simulink model "vx_vy_fixed_fusion_v2_5c_compile_harness"  (R2024a)
settings: Solver=FixedStepDiscrete  StartTime=0  StopTime=0.1  FixedStep=0.001  RelTol=1e-3
model workspace (MAT data in the model file):
  vy_v17_mode_code = 20
undefined symbols (not defined in the file or in its folder): vy_dynamic_ekf_v1_17
libraries: simulink x3
Description:
  | V2.5-C estimator-only compile harness. No CarSim or plant. Fusion weights [1/3 1/3 1/3] are TEST-ONLY, NOT SELECTED, NOT TUNED, NOT FROZEN. F feedback valid is fixed false and Vy_FW is not fed back.
settings Model: Creator=21180  LastModifiedBy=21180

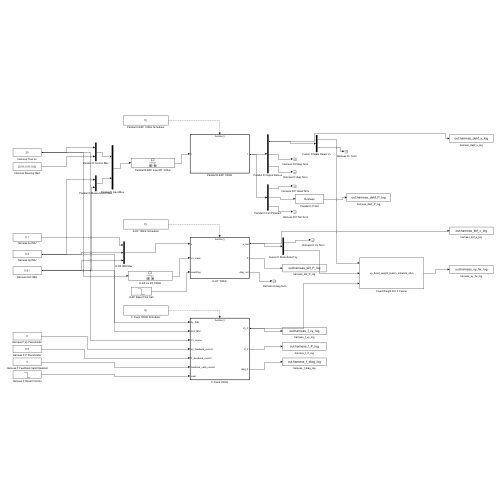
[thumbnail: Simulink's stored preview of the top-level diagram]
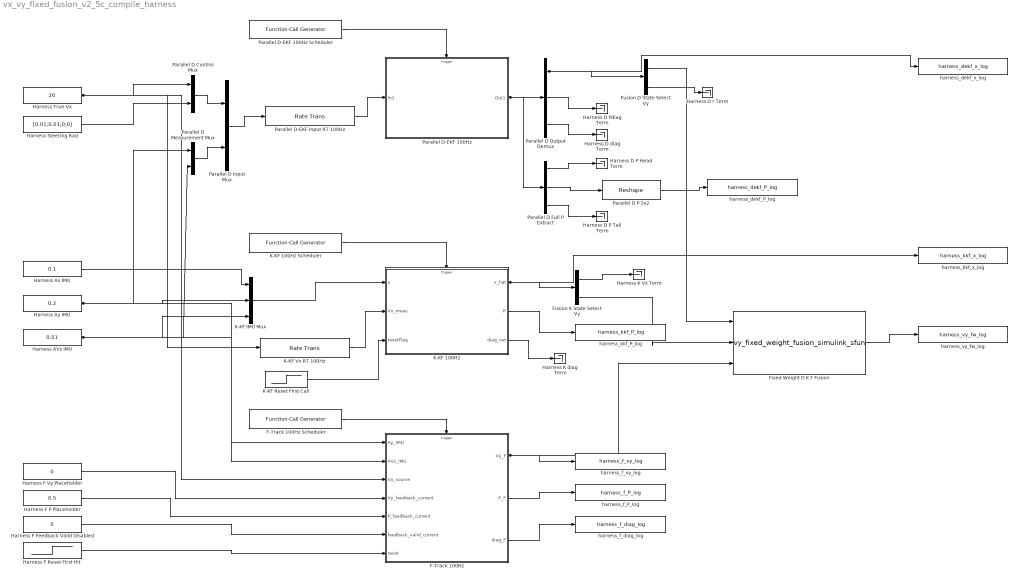
== system vx_vy_fixed_fusion_v2_5c_compile_harness ==
  F-Track 100Hz : Subsystem  TreatAsAtomicUnit=on
  F-Track 100Hz Scheduler : simulink/Ports & Subsystems/Function-Call Generator  sample_time=0.01  numberOfIterations=1  DisallowWideOutput=off
  Fixed Weight D K F Fusion : M-S-Function  FunctionName=vy_fixed_weight_fusion_simulink_sfun  Parameters=1/3,1/3,1/3
  Fusion D State Select Vy : Demux  Outputs=2
  Fusion K State Select Vy : Demux  Outputs=2
  Harness AVz IMU : Constant  Value=0.01  OutDataTypeStr=double  SampleTime=0.01
  Harness Ax IMU : Constant  Value=0.1  OutDataTypeStr=double  SampleTime=0.01
  Harness Ay IMU : Constant  Value=0.2  OutDataTypeStr=double  SampleTime=0.01
  Harness D P Head Term : Terminator
  Harness D P Tail Term : Terminator
  Harness D Pdiag Term : Terminator
  Harness D diag Term : Terminator
  Harness D r Term : Terminator
  Harness F Feedback Valid Disabled : Constant  Value=0  OutDataTypeStr=double  SampleTime=0.01
  Harness F P Placeholder : Constant  Value=0.5  OutDataTypeStr=double  SampleTime=0.01
  Harness F Reset First Hit : Step  Time=0.01  Before=1  After=0  SampleTime=0.01
  Harness F Vy Placeholder : Constant  Value=0  OutDataTypeStr=double  SampleTime=0.01
  Harness K Vx Term : Terminator
  Harness K diag Term : Terminator
  Harness Steering Rad : Constant  Value=[0.01;0.01;0;0]  OutDataTypeStr=double  SampleTime=0.01
  Harness True Vx : Constant  Value=20  OutDataTypeStr=double  SampleTime=0.001
  K-KF 100Hz : Subsystem  TreatAsAtomicUnit=on
  K-KF 100Hz Scheduler : simulink/Ports & Subsystems/Function-Call Generator  sample_time=0.01  numberOfIterations=1  DisallowWideOutput=off
  K-KF IMU Mux : Mux  Inputs=3
  K-KF Reset First Call : Step  Time=0.01  Before=1  After=0  SampleTime=0.01
  K-KF Vx RT 100Hz : RateTransition  OutPortSampleTime=0.01
  Parallel D Control Mux : Mux  Inputs=[1 4]
  Parallel D Full P Extract : Demux  Outputs=[45 4 20]
  Parallel D Input Mux : Mux  Inputs=[5 2]
  Parallel D Measurement Mux : Mux  Inputs=2
  Parallel D Output Demux : Demux  Outputs=[2 2 65]
  Parallel D P 2x2 : Reshape  OutputDimensionality=Customize  OutputDimensions=[2 2]
  Parallel D-EKF 100Hz : Subsystem  TreatAsAtomicUnit=on
  Parallel D-EKF 100Hz Scheduler : simulink/Ports & Subsystems/Function-Call Generator  sample_time=0.01  numberOfIterations=1  DisallowWideOutput=off
  Parallel D-EKF Input RT 100Hz : RateTransition  OutPortSampleTime=0.01
  harness_dekf_P_log : ToWorkspace  VariableName=harness_dekf_P_log  SaveFormat=Timeseries  SampleTime=-1
  harness_dekf_x_log : ToWorkspace  VariableName=harness_dekf_x_log  SaveFormat=Timeseries  SampleTime=-1
  harness_f_P_log : ToWorkspace  VariableName=harness_f_P_log  SaveFormat=Timeseries  SampleTime=-1
  harness_f_diag_log : ToWorkspace  VariableName=harness_f_diag_log  SaveFormat=Timeseries  SampleTime=-1
  harness_f_vy_log : ToWorkspace  VariableName=harness_f_vy_log  SaveFormat=Timeseries  SampleTime=-1
  harness_kkf_P_log : ToWorkspace  VariableName=harness_kkf_P_log  SaveFormat=Timeseries  SampleTime=-1
  harness_kkf_x_log : ToWorkspace  VariableName=harness_kkf_x_log  SaveFormat=Timeseries  SampleTime=-1
  harness_vy_fw_log : ToWorkspace  VariableName=harness_vy_fw_log  SaveFormat=Timeseries  SampleTime=-1
  wires:
  Harness True Vx/1 -> Parallel D Control Mux/1, K-KF Vx RT 100Hz/1, F-Track 100Hz/3(Vx_source)
  Harness Steering Rad/1 -> Parallel D Control Mux/2
  Harness Ay IMU/1 -> Parallel D Measurement Mux/1, K-KF IMU Mux/2, F-Track 100Hz/1(Ay_IMU)
  Harness AVz IMU/1 -> Parallel D Measurement Mux/2, K-KF IMU Mux/3, F-Track 100Hz/2(AVz_IMU)
  Parallel D Control Mux/1 -> Parallel D Input Mux/1
  Parallel D Measurement Mux/1 -> Parallel D Input Mux/2
  Parallel D Input Mux/1 -> Parallel D-EKF Input RT 100Hz/1
  Parallel D-EKF Input RT 100Hz/1 -> Parallel D-EKF 100Hz/1(In1)
  Parallel D-EKF 100Hz Scheduler/1 -> Parallel D-EKF 100Hz/Trigger
  Parallel D-EKF 100Hz/1(Out1) -> Parallel D Output Demux/1, Parallel D Full P Extract/1
  Parallel D Full P Extract/2 -> Parallel D P 2x2/1
  Harness Ax IMU/1 -> K-KF IMU Mux/1
  K-KF IMU Mux/1 -> K-KF 100Hz/1(u)
  K-KF Vx RT 100Hz/1 -> K-KF 100Hz/2(Vx_meas)
  K-KF Reset First Call/1 -> K-KF 100Hz/3(resetFlag)
  K-KF 100Hz Scheduler/1 -> K-KF 100Hz/Trigger
  Harness F Vy Placeholder/1 -> F-Track 100Hz/4(Vy_feedback_current)
  Harness F P Placeholder/1 -> F-Track 100Hz/5(P_feedback_current)
  Harness F Feedback Valid Disabled/1 -> F-Track 100Hz/6(feedback_valid_current)
  Harness F Reset First Hit/1 -> F-Track 100Hz/7(reset)
  F-Track 100Hz Scheduler/1 -> F-Track 100Hz/Trigger
  Parallel D Output Demux/1 -> Fusion D State Select Vy/1, harness_dekf_x_log/1
  K-KF 100Hz/1(x_hat) -> Fusion K State Select Vy/1, harness_kkf_x_log/1
  Fusion D State Select Vy/1 -> Fixed Weight D K F Fusion/1
  Fusion K State Select Vy/2 -> Fixed Weight D K F Fusion/2
  F-Track 100Hz/1(Vy_F) -> Fixed Weight D K F Fusion/3, harness_f_vy_log/1
  Parallel D P 2x2/1 -> harness_dekf_P_log/1
  K-KF 100Hz/2(P) -> harness_kkf_P_log/1
  F-Track 100Hz/2(P_F) -> harness_f_P_log/1
  F-Track 100Hz/3(diag_F) -> harness_f_diag_log/1
  Fixed Weight D K F Fusion/1 -> harness_vy_fw_log/1
  Parallel D Output Demux/2 -> Harness D Pdiag Term/1
  Parallel D Output Demux/3 -> Harness D diag Term/1
  Parallel D Full P Extract/1 -> Harness D P Head Term/1
  Parallel D Full P Extract/3 -> Harness D P Tail Term/1
  Fusion D State Select Vy/2 -> Harness D r Term/1
  Fusion K State Select Vy/1 -> Harness K Vx Term/1
  K-KF 100Hz/3(diag_out) -> Harness K diag Term/1

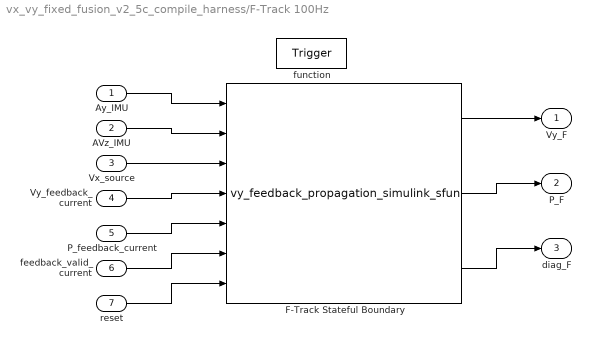
== system vx_vy_fixed_fusion_v2_5c_compile_harness/F-Track 100Hz ==
  Ay_IMU : Inport
  AVz_IMU : Inport  Port=2
  Vx_source : Inport  Port=3
  Vy_feedback_current : Inport  Port=4
  P_feedback_current : Inport  Port=5
  feedback_valid_current : Inport  Port=6
  reset : Inport  Port=7
  function : TriggerPort  TriggerType=function-call  VariantControl=(inherit)
  F-Track Stateful Boundary : M-S-Function  FunctionName=vy_feedback_propagation_simulink_sfun  Parameters=0.01,0,0.5,0.0025
  Vy_F : Outport
  P_F : Outport  Port=2
  diag_F : Outport  Port=3
  wires:
  Ay_IMU/1 -> F-Track Stateful Boundary/1
  AVz_IMU/1 -> F-Track Stateful Boundary/2
  Vx_source/1 -> F-Track Stateful Boundary/3
  Vy_feedback_current/1 -> F-Track Stateful Boundary/4
  P_feedback_current/1 -> F-Track Stateful Boundary/5
  feedback_valid_current/1 -> F-Track Stateful Boundary/6
  reset/1 -> F-Track Stateful Boundary/7
  F-Track Stateful Boundary/1 -> Vy_F/1
  F-Track Stateful Boundary/2 -> P_F/1
  F-Track Stateful Boundary/3 -> diag_F/1

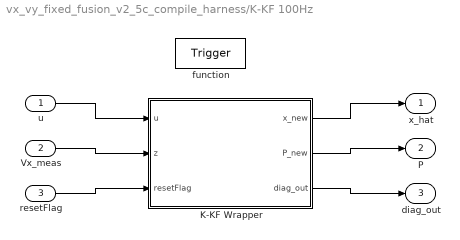
== system vx_vy_fixed_fusion_v2_5c_compile_harness/K-KF 100Hz ==
  u : Inport
  Vx_meas : Inport  Port=2
  resetFlag : Inport  Port=3
  function : TriggerPort  TriggerType=function-call  VariantControl=(inherit)
  K-KF Wrapper : MATLAB Function  TreatAsAtomicUnit=on
  x_hat : Outport
  P : Outport  Port=2
  diag_out : Outport  Port=3
  wires:
  K-KF Wrapper/3(diag_out) -> diag_out/1
  K-KF Wrapper/2(P_new) -> P/1
  K-KF Wrapper/1(x_new) -> x_hat/1
  resetFlag/1 -> K-KF Wrapper/3(resetFlag)
  Vx_meas/1 -> K-KF Wrapper/2(z)
  u/1 -> K-KF Wrapper/1(u)

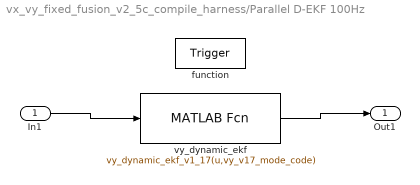
== system vx_vy_fixed_fusion_v2_5c_compile_harness/Parallel D-EKF 100Hz ==
  In1 : Inport
  function : TriggerPort  TriggerType=function-call  VariantControl=(inherit)
  vy_dynamic_ekf : MATLABFcn  MATLABFcn=vy_dynamic_ekf_v1_17(u,vy_v17_mode_code)  OutputDimensions=69
  Out1 : Outport
  wires:
  In1/1 -> vy_dynamic_ekf/1
  vy_dynamic_ekf/1 -> Out1/1

== matlab function vx_vy_fixed_fusion_v2_5c_compile_harness/K-KF 100Hz/K-KF Wrapper ==
  data: x_new output; u input; z input; resetFlag input; P_new output; diag_out output
function [x_new,P_new,diag_out] = kkf_wrapper(u,z,resetFlag)
%#codegen
[x_new,P_new,diag_out] = vy_kinematic_kf(u,z,resetFlag);
end
